simulink model "ee_580_project"  (R2020b)
settings: Solver=ode1  StartTime=0.0  StopTime=10.0  FixedStep=.05  RelTol=1e-3
values from neighbouring files (symbols this model uses):
  Aol = eye(4) + Ac*Ts    [KF_TEST_FPGA.m]    (also in kalman_filter_practice.m = sys_d.A)
  Bol = Bc*Ts    [KF_TEST_FPGA.m]    (also in kalman_filter_practice.m = sys_d.B)
  Col = Cc    [KF_TEST_FPGA.m]    (also in kalman_filter_practice.m = sys_d.C)
  L = 3e-3    (= 0.003)    [KF_TEST_FPGA.m]
libraries: simulink x2
settings Model: Creator=mcapuano  LastModifiedBy=mcapuano

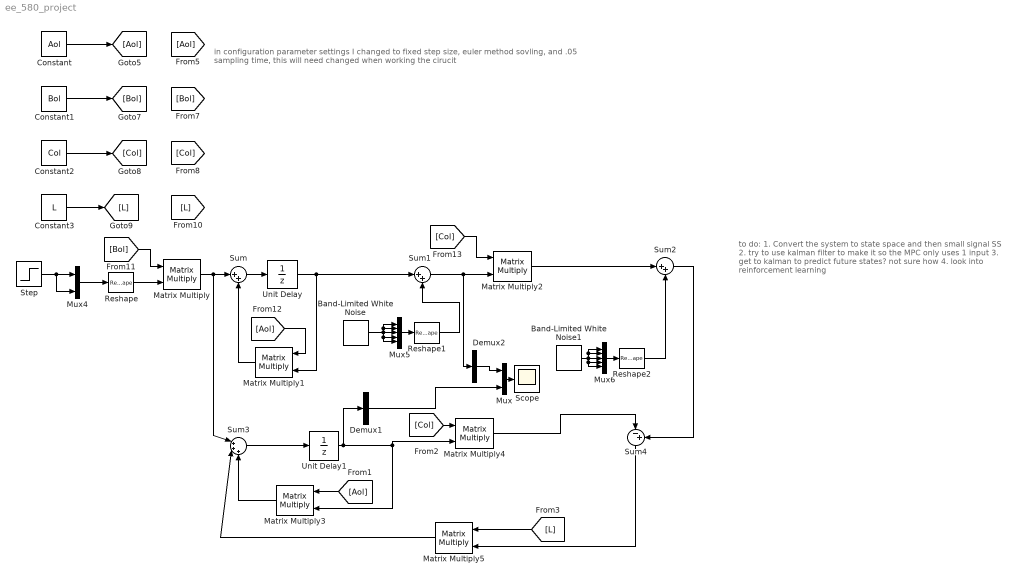
== system ee_580_project ==
  note: to do:
      | 1. Convert the system to state space and then small signal SS
      | 2. try to use kalman filter to make it so the MPC only uses 1 input
      | 3. get to kalman to predict future states? not sure how
      | 4. look into reinforcement learning
  note: in configuration parameter settings I changed to fixed step size, euler method sovling, and .05 sampling time, this will need changed when working the cirucit
  Band-Limited White Noise : simulink/Sources/Band-Limited White Noise  Cov=[0.1]  Ts=.05  seed=[23341]
  Band-Limited White Noise1 : simulink/Sources/Band-Limited White Noise  Cov=[0.1]  Ts=.05  seed=[23341]
  Constant : Constant  Value=Aol
  Constant1 : Constant  Value=Bol
  Constant2 : Constant  Value=Col
  Constant3 : Constant  Value=L
  Demux1 : Demux  Outputs=5
  Demux2 : Demux  Outputs=5
  Matrix Multiply{,1..5} (6 alike) : Product  Multiplication=Matrix(*)
  Mux : Mux  Inputs=2
  Mux4 : Mux  Inputs=2
  Mux5 : Mux  Inputs=5
  Mux6 : Mux  Inputs=5
  Reshape : Reshape  OutputDimensionality=Customize  OutputDimensions=[2,1]
  Reshape1 : Reshape  OutputDimensionality=Customize  OutputDimensions=[5,1]
  Reshape2 : Reshape  OutputDimensionality=Customize  OutputDimensions=[5,1]
  Scope : Scope
  Step : Step  SampleTime=0
  Sum : Sum  Inputs=|++
  Sum1 : Sum  Inputs=|++
  Sum2 : Sum  Inputs=|++
  Sum3 : Sum  Inputs=|+++
  Sum4 : Sum  Inputs=|-+
  Unit Delay : UnitDelay  SampleTime=-1  HasFrameUpgradeWarning=on
  Unit Delay1 : UnitDelay  SampleTime=-1  HasFrameUpgradeWarning=on
  wires:
  Constant/1 -> [Aol]
  Constant1/1 -> [Bol]
  Constant2/1 -> [Col]
  Constant3/1 -> [L]
  Step/1 -> Mux4/2, Mux4/1
  Mux4/1 -> Reshape/1
  Reshape/1 -> Matrix Multiply/2
  [Bol] -> Matrix Multiply/1
  Matrix Multiply/1 -> Sum3/1, Sum/1
  Sum/1 -> Unit Delay/1
  Unit Delay/1 -> Matrix Multiply1/2, Sum1/1
  [Aol] -> Matrix Multiply1/1
  Matrix Multiply1/1 -> Sum/2
  Sum1/1 -> Demux2/1, Matrix Multiply2/2
  Band-Limited White Noise/1 -> Mux5/2, Mux5/1, Mux5/5, Mux5/4, Mux5/3
  Mux5/1 -> Reshape1/1
  Reshape1/1 -> Sum1/2
  [Col] -> Matrix Multiply2/1
  Reshape2/1 -> Sum2/2
  Mux6/1 -> Reshape2/1
  Band-Limited White Noise1/1 -> Mux6/2, Mux6/1, Mux6/5, Mux6/4, Mux6/3
  Matrix Multiply2/1 -> Sum2/1
  Sum2/1 -> Sum4/2
  Sum3/1 -> Unit Delay1/1
  [Aol] -> Matrix Multiply3/1
  Unit Delay1/1 -> Demux1/1, Matrix Multiply3/2, Matrix Multiply4/2
  [Col] -> Matrix Multiply4/1
  Matrix Multiply4/1 -> Sum4/1
  [L] -> Matrix Multiply5/1
  Sum4/1 -> Matrix Multiply5/2
  Matrix Multiply3/1 -> Sum3/3
  Matrix Multiply5/1 -> Sum3/2
  Mux/1 -> Scope/1
  Demux2/3 -> Mux/1
  Demux1/3 -> Mux/2
